simulink model "trajectory_planning_dev"  (R2018b)
settings: Solver=ode2  StartTime=0.0  StopTime=inf  FixedStep=0.002  RelTol=1e-3  EnableMultiTasking=on
model workspace (MAT data in the model file):
  m = 1000
undefined symbols (not defined in the file or in its folder): tS
settings Model: DataDictionary=trajectory_planning_dev.sldd  PauseTimes=6.42  Creator=wischnewski  LastModifiedBy=ga25xiw
settings DataIOCC: SaveFormat=StructureWithTime  SaveOutput=off  SignalLogging=off  DSMLogging=off  SaveTime=off
settings OptimizationCC: BlockReduction=off  OptimizeBlockIOStorage=off  BufferReuse=off  GlobalBufferReuse=off  ExpressionFolding=off  LocalBlockOutputs=off  OptimizeDataStoreBuffers=off  BusAssignmentInplaceUpdate=off
settings HardwareCC: ProdBitPerPointer=32  ProdBitPerSizeT=32  ProdBitPerPtrDiffT=32  ProdLargestAtomicFloat=None  ProdWordSize=32  ProdLongLongMode=on  ProdHWDeviceType=Generic->32-bit x86 compatible
settings ModelReferenceCC: PropagateSignalLabelsOutOfModel=off
settings SFSimCC: SFSimEcho=off  SimUseLocalCustomCode=off
settings RTWCC: Description=Generic Real-Time Target  RTWUseLocalCustomCode=off  RTWCompilerOptimization=on
settings CodeAppCC: StateflowObjectComments=on
settings GRTTargetCC: TargetLangStandard=C89/C90 (ANSI)

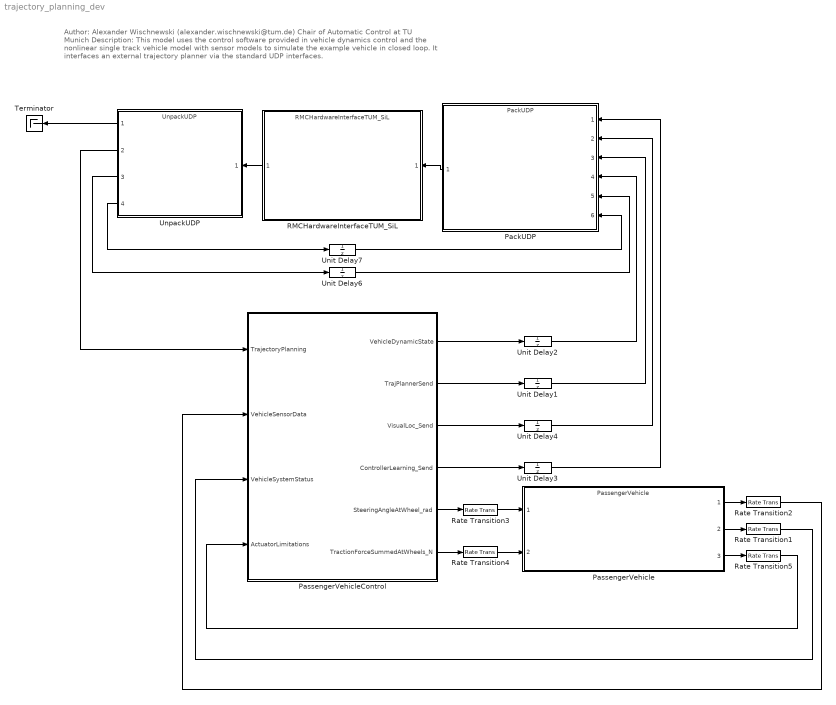
== system trajectory_planning_dev ==
  note: Author: Alexander Wischnewski (alexander.wischnewski@tum.de)
      | Chair of Automatic Control at TU Munich
      |
      | Description: This model uses the control software provided in vehicle dynamics control and the nonlinear single track vehicle model
      | with sensor models to simulate the example vehicle in closed loop. It interfaces an external trajectory planner via the standard UDP interfaces.
  PackUDP : ModelReference  ModelNameDialog=PackUDP  SimulationMode=Normal  ModelReferenceVersion=1.4127
  PassengerVehicle : ModelReference  ModelNameDialog=PassengerVehicle  SimulationMode=Normal  ModelReferenceVersion=1.714
  PassengerVehicleControl : Subsystem
  RMCHardwareInterfaceTUM_SiL : ModelReference  ModelNameDialog=RMCHardwareInterfaceTUM_SiL.slx  SimulationMode=Normal  ModelReferenceVersion=1.788
  Rate Transition{1..5} (5 alike) : RateTransition
  Terminator : Terminator
  Unit Delay{1..4,6..7} (6 alike) : UnitDelay  SampleTime=tS
  UnpackUDP : ModelReference  ModelNameDialog=UnpackUDP  SimulationMode=Normal  ModelReferenceVersion=1.4042
  wires:
  PackUDP/1 -> RMCHardwareInterfaceTUM_SiL/1
  RMCHardwareInterfaceTUM_SiL/1 -> UnpackUDP/1
  Unit Delay6/1 -> PackUDP/5
  UnpackUDP/3 -> Unit Delay6/1
  Unit Delay7/1 -> PackUDP/6
  UnpackUDP/4 -> Unit Delay7/1
  PassengerVehicle/2 -> Rate Transition1/1
  PassengerVehicle/3 -> Rate Transition5/1
  PassengerVehicle/1 -> Rate Transition2/1
  PassengerVehicleControl/5(SteeringAngleAtWheel_rad) -> Rate Transition3/1
  PassengerVehicleControl/6(TractionForceSummedAtWheels_N) -> Rate Transition4/1
  UnpackUDP/2 -> PassengerVehicleControl/1(TrajectoryPlanning)
  UnpackUDP/1 -> Terminator/1
  PassengerVehicleControl/2(TrajPlannerSend) -> Unit Delay1/1
  PassengerVehicleControl/1(VehicleDynamicState) -> Unit Delay2/1
  Unit Delay2/1 -> PackUDP/4
  Unit Delay1/1 -> PackUDP/3
  PassengerVehicleControl/3(VisualLoc_Send) -> Unit Delay4/1
  PassengerVehicleControl/4(ControllerLearning_Send) -> Unit Delay3/1
  Unit Delay4/1 -> PackUDP/2
  Unit Delay3/1 -> PackUDP/1
  Rate Transition2/1 -> PassengerVehicleControl/2(VehicleSensorData)
  Rate Transition1/1 -> PassengerVehicleControl/3(VehicleSystemStatus)
  Rate Transition5/1 -> PassengerVehicleControl/4(ActuatorLimitations)
  Rate Transition3/1 -> PassengerVehicle/1
  Rate Transition4/1 -> PassengerVehicle/2

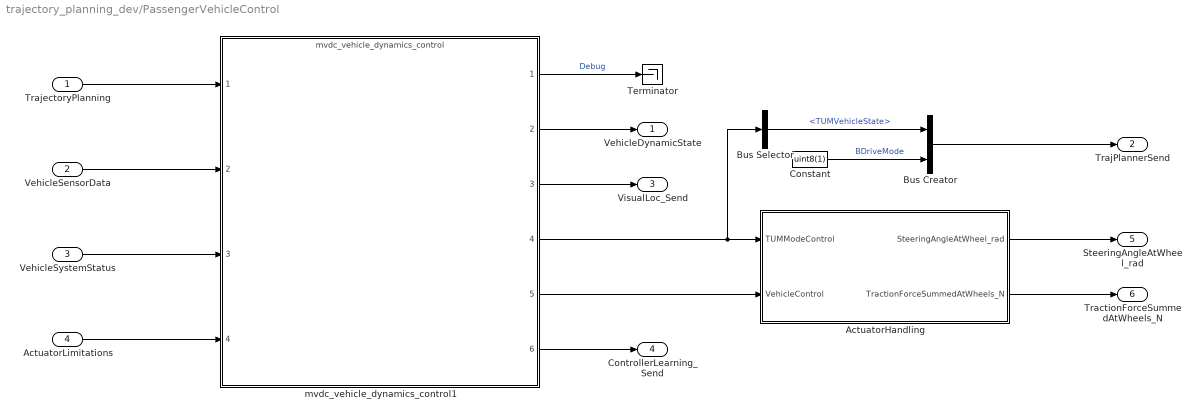
== system trajectory_planning_dev/PassengerVehicleControl ==
  TrajectoryPlanning : Inport
  VehicleSensorData : Inport  Port=2
  VehicleSystemStatus : Inport  Port=3
  ActuatorLimitations : Inport  Port=4
  ActuatorHandling : Subsystem
  Bus Creator : BusCreator  Inputs=2
  Bus Selector : BusSelector  OutputSignals=TUMVehicleState
  Constant : Constant  Value=uint8(1)
  Terminator : Terminator
  mvdc_vehicle_dynamics_control1 : ModelReference  ModelNameDialog=mvdc_vehicle_dynamics_control  SimulationMode=Normal  ModelReferenceVersion=1.757
  VehicleDynamicState : Outport
  TrajPlannerSend : Outport  Port=2
  VisualLoc_Send : Outport  Port=3
  ControllerLearning_Send : Outport  Port=4
  SteeringAngleAtWheel_rad : Outport  Port=5
  TractionForceSummedAtWheels_N : Outport  Port=6
  wires:
  mvdc_vehicle_dynamics_control1/1 -> Terminator/1  "Debug"
  VehicleSystemStatus/1 -> mvdc_vehicle_dynamics_control1/3
  ActuatorLimitations/1 -> mvdc_vehicle_dynamics_control1/4
  VehicleSensorData/1 -> mvdc_vehicle_dynamics_control1/2
  TrajectoryPlanning/1 -> mvdc_vehicle_dynamics_control1/1
  mvdc_vehicle_dynamics_control1/5 -> ActuatorHandling/2(VehicleControl)
  mvdc_vehicle_dynamics_control1/4 -> Bus Selector/1, ActuatorHandling/1(TUMModeControl)
  mvdc_vehicle_dynamics_control1/2 -> VehicleDynamicState/1
  ActuatorHandling/2(TractionForceSummedAtWheels_N) -> TractionForceSummedAtWheels_N/1
  ActuatorHandling/1(SteeringAngleAtWheel_rad) -> SteeringAngleAtWheel_rad/1
  Bus Selector/1 -> Bus Creator/1  "<TUMVehicleState>"
  Constant/1 -> Bus Creator/2  "BDriveMode"
  Bus Creator/1 -> TrajPlannerSend/1
  mvdc_vehicle_dynamics_control1/3 -> VisualLoc_Send/1
  mvdc_vehicle_dynamics_control1/6 -> ControllerLearning_Send/1

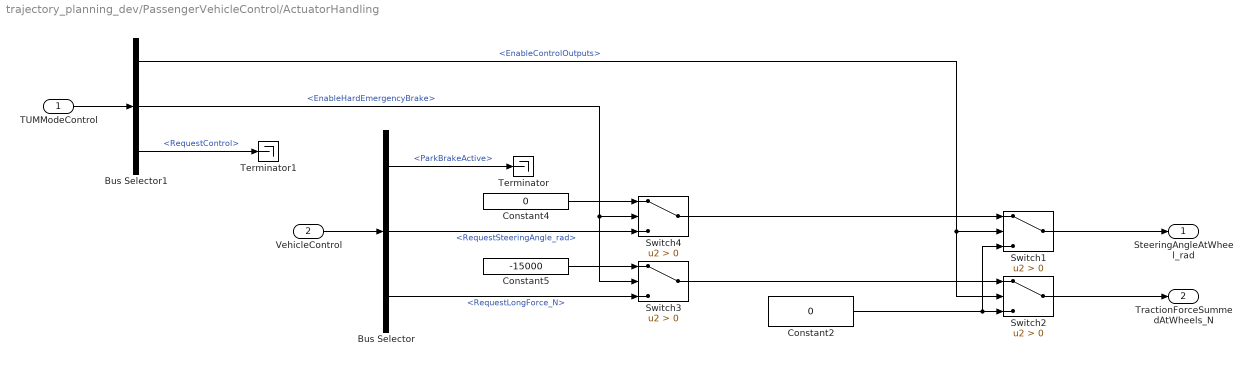
== system trajectory_planning_dev/PassengerVehicleControl/ActuatorHandling ==
  TUMModeControl : Inport  OutDataTypeStr=Bus: TUMModeControl
  VehicleControl : Inport  Port=2  OutDataTypeStr=Bus: VehicleControl
  Bus Selector : BusSelector  OutputSignals=ParkBrakeActive,RequestSteeringAngle_rad,RequestLongForce_N
  Bus Selector1 : BusSelector  OutputSignals=EnableControlOutputs,EnableHardEmergencyBrake,RequestControl
  Constant2 : Constant  Value=0
  Constant4 : Constant  Value=0
  Constant5 : Constant  Value=-15000
  Switch{1..4} (4 alike) : Switch  Criteria=u2 > Threshold
  Terminator : Terminator
  Terminator1 : Terminator
  SteeringAngleAtWheel_rad : Outport
  TractionForceSummedAtWheels_N : Outport  Port=2
  wires:
  Bus Selector1/1 -> Switch2/2, Switch1/2  "<EnableControlOutputs>"
  TUMModeControl/1 -> Bus Selector1/1
  Bus Selector/3 -> Switch3/3  "<RequestLongForce_N>"
  Constant2/1 -> Switch1/3, Switch2/3
  VehicleControl/1 -> Bus Selector/1
  Bus Selector/2 -> Switch4/3  "<RequestSteeringAngle_rad>"
  Constant4/1 -> Switch4/1
  Constant5/1 -> Switch3/1
  Bus Selector1/2 -> Switch3/2, Switch4/2  "<EnableHardEmergencyBrake>"
  Bus Selector/1 -> Terminator/1  "<ParkBrakeActive>"
  Bus Selector1/3 -> Terminator1/1  "<RequestControl>"
  Switch4/1 -> Switch1/1
  Switch3/1 -> Switch2/1
  Switch1/1 -> SteeringAngleAtWheel_rad/1
  Switch2/1 -> TractionForceSummedAtWheels_N/1
